simulink model "benign_PP"  (R2017a)
settings: Solver=FixedStepDiscrete  StartTime=0.0  StopTime=100  FixedStep=1  RelTol=1e-3
model workspace (MAT data in the model file):
  MCOS : class17 (value not decoded)
  compositionalMap : struct (value not decoded)
  isPreprocessedModel = 1
  MCOS : class17 (value not decoded)
  verificationResults : struct (value not decoded)
undefined symbols (not defined in the file or in its folder): contractAfterSimulation, contractBeforeSimulation, saveValidatorParameters
undefined symbols (not defined in the file): ContractBlock, ContractGuaranteeBlock, ContractValidatorBlock
libraries: simulink x436, CoCoSimSpecification x31
(part 3 of 3)

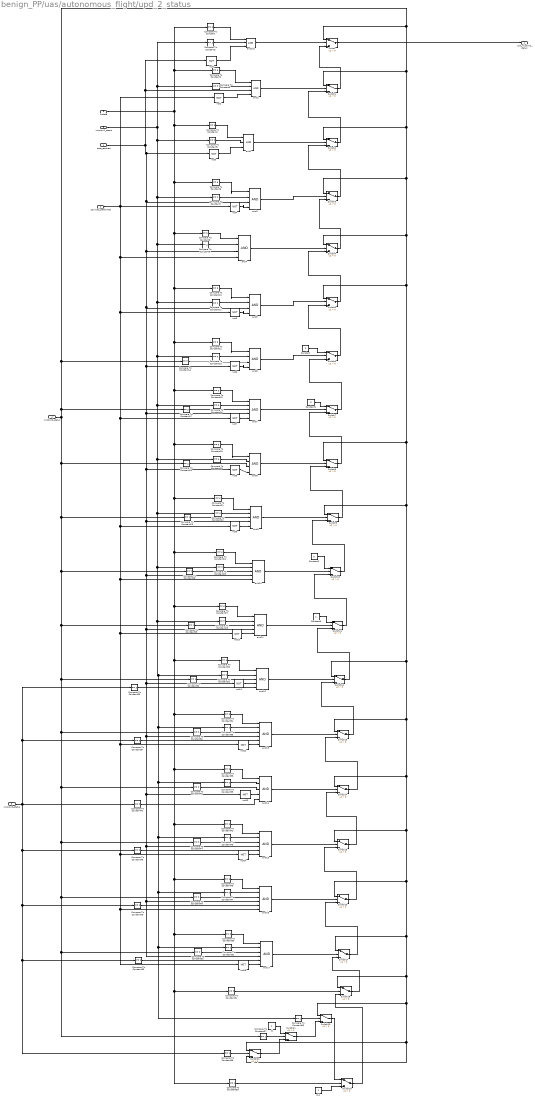
== system benign_PP/uas/autonomous_flight/upd_2_status ==
  dest_reached : Inport  OutDataTypeStr=boolean
  payload_performed : Inport  Port=2  OutDataTypeStr=boolean
  mission1_status : Inport  Port=3  OutDataTypeStr=int32
  mission2_status : Inport  Port=4  OutDataTypeStr=int32
  mission3_status : Inport  Port=5  OutDataTypeStr=int32
  mstate : Inport  Port=6  OutDataTypeStr=int32
  Compare To Constant{,2,4,6,8,10,12,15,18,21,24,27,30,34,38,42,46,50} (18 alike) : simulink/Logic and Bit Operations/Compare To Constant  relop===  const=6  OutDataTypeStr=boolean
  Compare To Constant{1,3,14,17,33,37,54} (7 alike) : simulink/Logic and Bit Operations/Compare To Constant  relop===  const=3  OutDataTypeStr=boolean
  Compare To Constant{5,7,9,11,20,23,26,29,41,45,49,53,56..58} (15 alike) : simulink/Logic and Bit Operations/Compare To Constant  relop===  const=2  OutDataTypeStr=boolean
  Compare To Constant{13,16,19,22,25,28,31..32,35..36,39..40,43..44,47..48,51..52} (18 alike) : simulink/Logic and Bit Operations/Compare To Constant  relop===  const=0  OutDataTypeStr=boolean
  Compare To Constant55 : simulink/Logic and Bit Operations/Compare To Constant  relop===  const=4  OutDataTypeStr=boolean
  Constant : Constant  Value=2  OutDataTypeStr=int32
  Constant1 : Constant  Value=2  OutDataTypeStr=int32
  Constant2 : Constant  Value=0  OutDataTypeStr=int32
  Constant3 : Constant  OutDataTypeStr=int32
  Switch{,2..22} (22 alike) : Switch  Criteria=u2 > Threshold
  Switch1 : Switch  Criteria=u2 > Threshold  OutDataTypeStr=int32
  and1 : Logic  Inputs=3  IconShape=distinctive  AllPortsSameDT=off  OutDataTypeStr=boolean
  and{7,9..12,14} (6 alike) : Logic  Inputs=5  IconShape=distinctive  AllPortsSameDT=off  OutDataTypeStr=boolean
  and101 : Logic  Inputs=3  IconShape=distinctive  AllPortsSameDT=off  OutDataTypeStr=boolean
  and{13,15..17} (4 alike) : Logic  Inputs=6  IconShape=distinctive  AllPortsSameDT=off  OutDataTypeStr=boolean
  and{2..6,8} (6 alike) : Logic  Inputs=4  IconShape=distinctive  AllPortsSameDT=off  OutDataTypeStr=boolean
  c1 : Constant  OutDataTypeStr=int32
  c11 : Constant  OutDataTypeStr=int32
  not{1..15} (15 alike) : Logic  Operator=NOT  Inputs=3  IconShape=distinctive  AllPortsSameDT=off  OutDataTypeStr=boolean
  upd_mission2_status : Outport  OutDataTypeStr=int32
  wires:
  c11/1 -> Switch19/3
  Switch/1 -> upd_mission2_status/1
  and101/1 -> Switch/2
  Compare To Constant/1 -> and101/1
  Compare To Constant1/1 -> and101/2
  not1/1 -> and101/3
  Compare To Constant3/1 -> and2/2
  Compare To Constant2/1 -> and2/1
  Switch1/1 -> Switch/3
  and2/1 -> Switch1/2
  not2/1 -> and2/4
  Switch2/1 -> Switch1/3
  Compare To Constant4/1 -> and1/1
  Compare To Constant5/1 -> and1/2
  and1/1 -> Switch2/2
  not3/1 -> and1/3
  and3/1 -> Switch3/2
  Compare To Constant7/1 -> and3/2
  Switch3/1 -> Switch2/3
  Compare To Constant6/1 -> and3/1
  not4/1 -> and3/4
  Compare To Constant8/1 -> and4/1
  and4/1 -> Switch4/2
  Compare To Constant9/1 -> and4/2
  Switch4/1 -> Switch3/3
  Compare To Constant10/1 -> and5/1
  Compare To Constant11/1 -> and5/2
  and5/1 -> Switch5/2
  not5/1 -> and5/4
  Switch5/1 -> Switch4/3
  Compare To Constant13/1 -> and6/2
  Compare To Constant12/1 -> and6/1
  not6/1 -> and6/4
  Switch6/1 -> Switch5/3
  and6/1 -> Switch6/2
  Compare To Constant14/1 -> and6/3
  Compare To Constant17/1 -> and7/3
  and7/1 -> Switch7/2
  Compare To Constant16/1 -> and7/2
  Compare To Constant15/1 -> and7/1
  Switch7/1 -> Switch6/3
  not7/1 -> and7/5
  Compare To Constant18/1 -> and8/1
  Compare To Constant20/1 -> and8/3
  and8/1 -> Switch8/2
  Switch8/1 -> Switch7/3
  Compare To Constant19/1 -> and8/2
  not8/1 -> and8/4
  Switch9/1 -> Switch8/3
  Compare To Constant21/1 -> and9/1
  Compare To Constant23/1 -> and9/3
  and9/1 -> Switch9/2
  Compare To Constant22/1 -> and9/2
  not9/1 -> and9/5
  Switch10/1 -> Switch9/3
  and10/1 -> Switch10/2
  Compare To Constant24/1 -> and10/1
  Compare To Constant26/1 -> and10/3
  Compare To Constant25/1 -> and10/2
  Switch11/1 -> Switch10/3
  Compare To Constant29/1 -> and11/3
  and11/1 -> Switch11/2
  Compare To Constant28/1 -> and11/2
  Compare To Constant27/1 -> and11/1
  not10/1 -> and11/5
  Compare To Constant30/1 -> and12/1
  Switch12/1 -> Switch11/3
  Compare To Constant31/1 -> and12/2
  and12/1 -> Switch12/2
  Compare To Constant32/1 -> and12/3
  not11/1 -> and12/4
  Compare To Constant33/1 -> and12/5
  Switch13/1 -> Switch12/3
  Compare To Constant37/1 -> and13/5
  and13/1 -> Switch13/2
  Compare To Constant34/1 -> and13/1
  Compare To Constant35/1 -> and13/2
  Compare To Constant36/1 -> and13/3
  not12/1 -> and13/6
  Compare To Constant40/1 -> and14/3
  Compare To Constant39/1 -> and14/2
  Compare To Constant38/1 -> and14/1
  Compare To Constant41/1 -> and14/5
  Switch14/1 -> Switch13/3
  and14/1 -> Switch14/2
  not13/1 -> and14/4
  and15/1 -> Switch15/2
  Compare To Constant45/1 -> and15/5
  Compare To Constant44/1 -> and15/3
  Switch15/1 -> Switch14/3
  not14/1 -> and15/6
  Compare To Constant42/1 -> and15/1
  Compare To Constant43/1 -> and15/2
  Switch16/1 -> Switch15/3
  Compare To Constant46/1 -> and16/1
  and16/1 -> Switch16/2
  Compare To Constant48/1 -> and16/3
  Compare To Constant47/1 -> and16/2
  Compare To Constant49/1 -> and16/5
  and17/1 -> Switch17/2
  Compare To Constant51/1 -> and17/2
  dest_reached/1 -> and2/3, not1/1, and9/4, and16/4, and17/4, and15/4, not13/1, and13/4, not11/1, and11/4, and10/4, not8/1, and7/4, not6/1, and5/3, and4/3, and3/3, not3/1
  Compare To Constant53/1 -> and17/5
  Compare To Constant50/1 -> and17/1
  mission1_status/1 -> Compare To Constant7/1, Compare To Constant56/1, Compare To Constant51/1, Compare To Constant47/1, Compare To Constant43/1, Compare To Constant39/1, Compare To Constant35/1, Compare To Constant31/1, Compare To Constant28/1, Compare To Constant25/1, Compare To Constant22/1, Compare To Constant19/1, Compare To Constant16/1, Compare To Constant13/1, Compare To Constant11/1, Compare To Constant9/1, Compare To Constant5/1, Compare To Constant3/1, Compare To Constant1/1
  Compare To Constant52/1 -> and17/3
  Switch17/1 -> Switch16/3
  not15/1 -> and17/6
  Switch18/1 -> Switch17/3
  Compare To Constant54/1 -> Switch18/2
  Switch19/1 -> Switch18/3
  mstate/1 -> Compare To Constant6/1, Compare To Constant12/1, Compare To Constant27/1, Compare To Constant55/1, Compare To Constant54/1, Compare To Constant50/1, Compare To Constant46/1, Compare To Constant42/1, Compare To Constant38/1, Compare To Constant34/1, Compare To Constant30/1, Compare To Constant24/1, Compare To Constant21/1, Compare To Constant18/1, Compare To Constant15/1, Compare To Constant10/1, Compare To Constant8/1, Compare To Constant4/1, Compare To Constant2/1, Compare To Constant/1
  Compare To Constant55/1 -> Switch19/2
  Compare To Constant56/1 -> Switch20/2
  mission2_status/1 -> Switch/1, Switch1/1, Switch2/1, Switch3/1, Switch4/1, Switch5/1, Switch8/1, Switch9/1, Switch12/1, Switch13/1, Switch14/1, Switch15/1, Switch16/1, Switch17/1, Switch18/1, Switch22/1, Switch22/3, Switch20/1, Compare To Constant14/1, Compare To Constant17/1, Compare To Constant57/1, Compare To Constant52/1, Compare To Constant48/1, Compare To Constant44/1, Compare To Constant40/1, Compare To Constant36/1, Compare To Constant32/1, Compare To Constant29/1, Compare To Constant26/1, Compare To Constant23/1, Compare To Constant20/1
  Switch20/1 -> Switch19/1
  Compare To Constant57/1 -> Switch21/2
  Switch21/1 -> Switch20/3
  Compare To Constant58/1 -> Switch22/2
  Switch22/1 -> Switch21/3
  mission3_status/1 -> Compare To Constant33/1, Compare To Constant37/1, Compare To Constant49/1, Compare To Constant58/1, Compare To Constant53/1, Compare To Constant45/1, Compare To Constant41/1
  payload_performed/1 -> not2/1, not15/1, and16/6, not14/1, not12/1, not10/1, and10/5, not9/1, not7/1, not5/1, and4/4, not4/1
  Constant1/1 -> Switch7/1
  Constant/1 -> Switch6/1
  Constant2/1 -> Switch10/1
  Constant3/1 -> Switch11/1
  c1/1 -> Switch21/1

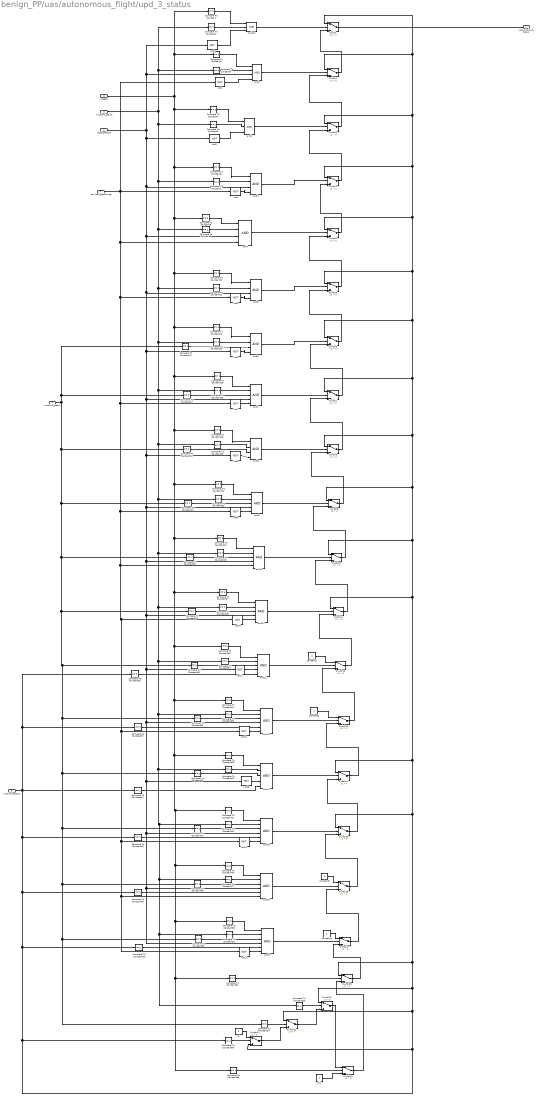
== system benign_PP/uas/autonomous_flight/upd_3_status ==
  dest_reached : Inport  OutDataTypeStr=boolean
  payload_performed : Inport  Port=2  OutDataTypeStr=boolean
  mission1_status : Inport  Port=3  OutDataTypeStr=int32
  mission2_status : Inport  Port=4  OutDataTypeStr=int32
  mission3_status : Inport  Port=5  OutDataTypeStr=int32
  mstate : Inport  Port=6  OutDataTypeStr=int32
  Compare To Constant{,2,4,6,8,10,12,15,18,21,24,27,30,34,38,42,46,50} (18 alike) : simulink/Logic and Bit Operations/Compare To Constant  relop===  const=6  OutDataTypeStr=boolean
  Compare To Constant{1,3,14,17,33,37,54} (7 alike) : simulink/Logic and Bit Operations/Compare To Constant  relop===  const=3  OutDataTypeStr=boolean
  Compare To Constant{5,7,9,11,20,23,26,29,41,45,49,53,56..58} (15 alike) : simulink/Logic and Bit Operations/Compare To Constant  relop===  const=2  OutDataTypeStr=boolean
  Compare To Constant{13,16,19,22,25,28,31..32,35..36,39..40,43..44,47..48,51..52} (18 alike) : simulink/Logic and Bit Operations/Compare To Constant  relop===  const=0  OutDataTypeStr=boolean
  Compare To Constant55 : simulink/Logic and Bit Operations/Compare To Constant  relop===  const=4  OutDataTypeStr=boolean
  Constant1 : Constant  Value=2  OutDataTypeStr=int32
  Constant2 : Constant  Value=2  OutDataTypeStr=int32
  Constant3 : Constant  Value=0  OutDataTypeStr=int32
  Constant4 : Constant  OutDataTypeStr=int32
  Switch : Switch  Criteria=u2 > Threshold  OutDataTypeStr=int32
  Switch{1..22} (22 alike) : Switch  Criteria=u2 > Threshold
  and1 : Logic  Inputs=3  IconShape=distinctive  AllPortsSameDT=off  OutDataTypeStr=boolean
  and{7,9..12,14} (6 alike) : Logic  Inputs=5  IconShape=distinctive  AllPortsSameDT=off  OutDataTypeStr=boolean
  and101 : Logic  Inputs=3  IconShape=distinctive  AllPortsSameDT=off  OutDataTypeStr=boolean
  and{13,15..17} (4 alike) : Logic  Inputs=6  IconShape=distinctive  AllPortsSameDT=off  OutDataTypeStr=boolean
  and{2..6,8} (6 alike) : Logic  Inputs=4  IconShape=distinctive  AllPortsSameDT=off  OutDataTypeStr=boolean
  c1 : Constant  OutDataTypeStr=int32
  c11 : Constant  OutDataTypeStr=int32
  not{1..15} (15 alike) : Logic  Operator=NOT  Inputs=3  IconShape=distinctive  AllPortsSameDT=off  OutDataTypeStr=boolean
  upd_mission3_status : Outport  OutDataTypeStr=int32
  wires:
  mission3_status/1 -> Compare To Constant41/1, Compare To Constant45/1, Compare To Constant53/1, Switch22/3, Switch21/1, Switch20/1, Switch18/1, Switch15/1, Switch14/1, Switch11/1, Switch10/1, Switch9/1, Switch8/1, Switch7/1, Switch6/1, Switch5/1, Switch4/1, Switch3/1, Switch2/1, Switch1/1, Switch/1, Compare To Constant58/1, Compare To Constant49/1, Compare To Constant37/1, Compare To Constant33/1
  payload_performed/1 -> not4/1, and4/4, not5/1, not7/1, not9/1, and10/5, not10/1, not12/1, not14/1, and16/6, not15/1, not2/1
  Switch22/1 -> Switch21/3
  Compare To Constant58/1 -> Switch22/2
  Switch21/1 -> Switch20/3
  Compare To Constant57/1 -> Switch21/2
  Switch20/1 -> Switch19/1
  mission2_status/1 -> Compare To Constant20/1, Compare To Constant23/1, Compare To Constant26/1, Compare To Constant29/1, Compare To Constant32/1, Compare To Constant36/1, Compare To Constant40/1, Compare To Constant44/1, Compare To Constant48/1, Compare To Constant52/1, Compare To Constant57/1, Compare To Constant17/1, Compare To Constant14/1
  Compare To Constant56/1 -> Switch20/2
  Compare To Constant55/1 -> Switch19/2
  mstate/1 -> Compare To Constant/1, Compare To Constant2/1, Compare To Constant4/1, Compare To Constant8/1, Compare To Constant10/1, Compare To Constant15/1, Compare To Constant18/1, Compare To Constant21/1, Compare To Constant24/1, Compare To Constant30/1, Compare To Constant34/1, Compare To Constant38/1, Compare To Constant42/1, Compare To Constant46/1, Compare To Constant50/1, Compare To Constant54/1, Compare To Constant55/1, Compare To Constant27/1, Compare To Constant12/1, Compare To Constant6/1
  Switch19/1 -> Switch18/3
  Compare To Constant54/1 -> Switch18/2
  Switch18/1 -> Switch17/3
  not15/1 -> and17/6
  Switch17/1 -> Switch16/3
  Compare To Constant52/1 -> and17/3
  mission1_status/1 -> Compare To Constant1/1, Compare To Constant3/1, Compare To Constant5/1, Compare To Constant9/1, Compare To Constant11/1, Compare To Constant13/1, Compare To Constant16/1, Compare To Constant19/1, Compare To Constant22/1, Compare To Constant25/1, Compare To Constant28/1, Compare To Constant31/1, Compare To Constant35/1, Compare To Constant39/1, Compare To Constant43/1, Compare To Constant47/1, Compare To Constant51/1, Compare To Constant56/1, Compare To Constant7/1
  Compare To Constant50/1 -> and17/1
  Compare To Constant53/1 -> and17/5
  dest_reached/1 -> not3/1, and3/3, and4/3, and5/3, not6/1, and7/4, not8/1, and10/4, and11/4, not11/1, and13/4, not13/1, and15/4, and17/4, and16/4, and9/4, not1/1, and2/3
  Compare To Constant51/1 -> and17/2
  and17/1 -> Switch17/2
  Compare To Constant49/1 -> and16/5
  Compare To Constant47/1 -> and16/2
  Compare To Constant48/1 -> and16/3
  and16/1 -> Switch16/2
  Compare To Constant46/1 -> and16/1
  Switch16/1 -> Switch15/3
  Compare To Constant43/1 -> and15/2
  Compare To Constant42/1 -> and15/1
  not14/1 -> and15/6
  Switch15/1 -> Switch14/3
  Compare To Constant44/1 -> and15/3
  Compare To Constant45/1 -> and15/5
  and15/1 -> Switch15/2
  not13/1 -> and14/4
  and14/1 -> Switch14/2
  Switch14/1 -> Switch13/3
  Compare To Constant41/1 -> and14/5
  Compare To Constant38/1 -> and14/1
  Compare To Constant39/1 -> and14/2
  Compare To Constant40/1 -> and14/3
  not12/1 -> and13/6
  Compare To Constant36/1 -> and13/3
  Compare To Constant35/1 -> and13/2
  Compare To Constant34/1 -> and13/1
  and13/1 -> Switch13/2
  Compare To Constant37/1 -> and13/5
  Switch13/1 -> Switch12/3
  Compare To Constant33/1 -> and12/5
  not11/1 -> and12/4
  Compare To Constant32/1 -> and12/3
  and12/1 -> Switch12/2
  Compare To Constant31/1 -> and12/2
  Switch12/1 -> Switch11/3
  Compare To Constant30/1 -> and12/1
  not10/1 -> and11/5
  Compare To Constant27/1 -> and11/1
  Compare To Constant28/1 -> and11/2
  and11/1 -> Switch11/2
  Compare To Constant29/1 -> and11/3
  Switch11/1 -> Switch10/3
  Compare To Constant25/1 -> and10/2
  Compare To Constant26/1 -> and10/3
  Compare To Constant24/1 -> and10/1
  and10/1 -> Switch10/2
  Switch10/1 -> Switch9/3
  not9/1 -> and9/5
  Compare To Constant22/1 -> and9/2
  and9/1 -> Switch9/2
  Compare To Constant23/1 -> and9/3
  Compare To Constant21/1 -> and9/1
  Switch9/1 -> Switch8/3
  not8/1 -> and8/4
  Compare To Constant19/1 -> and8/2
  Switch8/1 -> Switch7/3
  and8/1 -> Switch8/2
  Compare To Constant20/1 -> and8/3
  Compare To Constant18/1 -> and8/1
  not7/1 -> and7/5
  Switch7/1 -> Switch6/3
  Compare To Constant15/1 -> and7/1
  Compare To Constant16/1 -> and7/2
  and7/1 -> Switch7/2
  Compare To Constant17/1 -> and7/3
  Compare To Constant14/1 -> and6/3
  and6/1 -> Switch6/2
  Switch6/1 -> Switch5/3
  not6/1 -> and6/4
  Compare To Constant12/1 -> and6/1
  Compare To Constant13/1 -> and6/2
  Switch5/1 -> Switch4/3
  not5/1 -> and5/4
  and5/1 -> Switch5/2
  Compare To Constant11/1 -> and5/2
  Compare To Constant10/1 -> and5/1
  Switch4/1 -> Switch3/3
  Compare To Constant9/1 -> and4/2
  and4/1 -> Switch4/2
  Compare To Constant8/1 -> and4/1
  not4/1 -> and3/4
  Compare To Constant6/1 -> and3/1
  Switch3/1 -> Switch2/3
  Compare To Constant7/1 -> and3/2
  and3/1 -> Switch3/2
  not3/1 -> and1/3
  and1/1 -> Switch2/2
  Compare To Constant5/1 -> and1/2
  Compare To Constant4/1 -> and1/1
  Switch2/1 -> Switch1/3
  not2/1 -> and2/4
  and2/1 -> Switch1/2
  Switch1/1 -> Switch/3
  Compare To Constant2/1 -> and2/1
  Compare To Constant3/1 -> and2/2
  not1/1 -> and101/3
  Compare To Constant1/1 -> and101/2
  Compare To Constant/1 -> and101/1
  and101/1 -> Switch/2
  Switch/1 -> upd_mission3_status/1
  c11/1 -> Switch19/3
  Constant1/1 -> Switch12/1
  Constant2/1 -> Switch13/1
  Constant3/1 -> Switch16/1
  Constant4/1 -> Switch17/1
  c1/1 -> Switch22/1

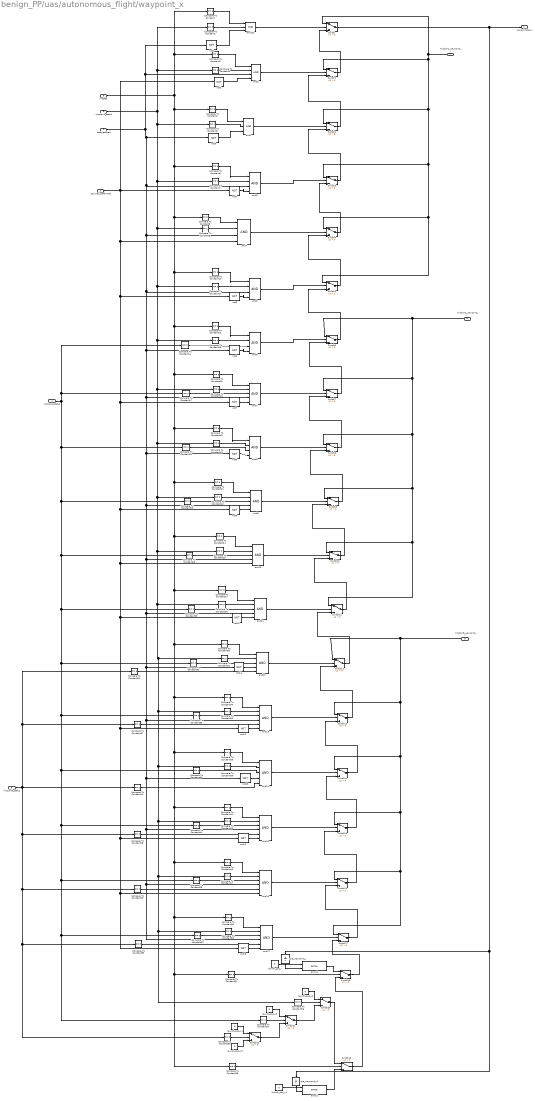
== system benign_PP/uas/autonomous_flight/waypoint_x ==
  dest_reached : Inport  OutDataTypeStr=boolean
  payload_performed : Inport  Port=2  OutDataTypeStr=boolean
  mission1_status : Inport  Port=3  OutDataTypeStr=int32
  mission2_status : Inport  Port=4  OutDataTypeStr=int32
  mission3_status : Inport  Port=5  OutDataTypeStr=int32
  mstate : Inport  Port=6  OutDataTypeStr=int32
  mission1_waypoint_x : Inport  Port=7  OutDataTypeStr=int32
  mission2_waypoint_x : Inport  Port=8  OutDataTypeStr=int32
  mission3_waypoint_x : Inport  Port=9  OutDataTypeStr=int32
  Compare To Constant{,2,4,6,8,10,12,15,18,21,24,27,30,34,38,42,46,50} (18 alike) : simulink/Logic and Bit Operations/Compare To Constant  relop===  const=6  OutDataTypeStr=boolean
  Compare To Constant{1,3,14,17,33,37,54} (7 alike) : simulink/Logic and Bit Operations/Compare To Constant  relop===  const=3  OutDataTypeStr=boolean
  Compare To Constant{5,7,9,11,20,23,26,29,41,45,49,53,56..58} (15 alike) : simulink/Logic and Bit Operations/Compare To Constant  relop===  const=2  OutDataTypeStr=boolean
  Compare To Constant{13,16,19,22,25,28,31..32,35..36,39..40,43..44,47..48,51..52} (18 alike) : simulink/Logic and Bit Operations/Compare To Constant  relop===  const=0  OutDataTypeStr=boolean
  Compare To Constant55 : simulink/Logic and Bit Operations/Compare To Constant  relop===  const=4  OutDataTypeStr=boolean
  Switch{,1..22} (23 alike) : Switch  Criteria=u2 > Threshold
  and1 : Logic  Inputs=3  IconShape=distinctive  AllPortsSameDT=off  OutDataTypeStr=boolean
  and{7,9..12,14} (6 alike) : Logic  Inputs=5  IconShape=distinctive  AllPortsSameDT=off  OutDataTypeStr=boolean
  and101 : Logic  Inputs=3  IconShape=distinctive  AllPortsSameDT=off  OutDataTypeStr=boolean
  and{13,15..17} (4 alike) : Logic  Inputs=6  IconShape=distinctive  AllPortsSameDT=off  OutDataTypeStr=boolean
  and{2..6,8} (6 alike) : Logic  Inputs=4  IconShape=distinctive  AllPortsSameDT=off  OutDataTypeStr=boolean
  arrow1 : CoCoSimSpecification/arrow  LustreOperatorBlock=ArrowOperator
      settings: SourceProductName=CoCoSim Specification
  arrow2 : CoCoSimSpecification/arrow  LustreOperatorBlock=ArrowOperator
      settings: SourceProductName=CoCoSim Specification
  launch_pos_x{,1..5} (6 alike) : Constant  Value=0  OutDataTypeStr=int32
  not{1..15} (15 alike) : Logic  Operator=NOT  Inputs=3  IconShape=distinctive  AllPortsSameDT=off  OutDataTypeStr=boolean
  pre_waypoint_x : UnitDelay  SampleTime=-1
  pre_waypoint_x1 : UnitDelay  SampleTime=-1
  waypointPos_x : Outport  OutDataTypeStr=int32
  wires:
  launch_pos_x5/1 -> Switch22/3
  mission3_status/1 -> Compare To Constant41/1, Compare To Constant45/1, Compare To Constant53/1, Compare To Constant58/1, Compare To Constant49/1, Compare To Constant37/1, Compare To Constant33/1
  launch_pos_x4/1 -> Switch22/1
  Switch22/1 -> Switch21/3
  Compare To Constant58/1 -> Switch22/2
  Switch21/1 -> Switch20/3
  Compare To Constant57/1 -> Switch21/2
  launch_pos_x3/1 -> Switch21/1
  Switch20/1 -> Switch19/1
  launch_pos_x2/1 -> Switch20/1
  Compare To Constant56/1 -> Switch20/2
  Compare To Constant55/1 -> Switch19/2
  mstate/1 -> Compare To Constant/1, Compare To Constant2/1, Compare To Constant4/1, Compare To Constant8/1, Compare To Constant10/1, Compare To Constant15/1, Compare To Constant18/1, Compare To Constant21/1, Compare To Constant24/1, Compare To Constant30/1, Compare To Constant34/1, Compare To Constant38/1, Compare To Constant42/1, Compare To Constant46/1, Compare To Constant50/1, Compare To Constant54/1, Compare To Constant55/1, Compare To Constant27/1, Compare To Constant12/1, Compare To Constant6/1
  Switch19/1 -> Switch18/3
  Compare To Constant54/1 -> Switch18/2
  Switch18/1 -> Switch17/3
  not15/1 -> and17/6
  Switch17/1 -> Switch16/3
  Compare To Constant52/1 -> and17/3
  mission1_status/1 -> Compare To Constant1/1, Compare To Constant3/1, Compare To Constant5/1, Compare To Constant9/1, Compare To Constant11/1, Compare To Constant13/1, Compare To Constant16/1, Compare To Constant19/1, Compare To Constant22/1, Compare To Constant25/1, Compare To Constant28/1, Compare To Constant31/1, Compare To Constant35/1, Compare To Constant39/1, Compare To Constant43/1, Compare To Constant47/1, Compare To Constant51/1, Compare To Constant56/1, Compare To Constant7/1
  Compare To Constant50/1 -> and17/1
  Compare To Constant53/1 -> and17/5
  dest_reached/1 -> not3/1, and3/3, and4/3, and5/3, not6/1, and7/4, not8/1, and10/4, and11/4, not11/1, and13/4, not13/1, and15/4, and17/4, and16/4, and9/4, not1/1, and2/3
  mission2_status/1 -> Compare To Constant20/1, Compare To Constant23/1, Compare To Constant26/1, Compare To Constant29/1, Compare To Constant32/1, Compare To Constant36/1, Compare To Constant40/1, Compare To Constant44/1, Compare To Constant48/1, Compare To Constant52/1, Compare To Constant57/1, Compare To Constant17/1, Compare To Constant14/1
  Compare To Constant51/1 -> and17/2
  payload_performed/1 -> not4/1, and4/4, not5/1, not7/1, not9/1, and10/5, not10/1, not12/1, not14/1, and16/6, not15/1, not2/1
  and17/1 -> Switch17/2
  Compare To Constant49/1 -> and16/5
  Compare To Constant47/1 -> and16/2
  Compare To Constant48/1 -> and16/3
  and16/1 -> Switch16/2
  Compare To Constant46/1 -> and16/1
  Switch16/1 -> Switch15/3
  Compare To Constant43/1 -> and15/2
  Compare To Constant42/1 -> and15/1
  not14/1 -> and15/6
  Switch15/1 -> Switch14/3
  Compare To Constant44/1 -> and15/3
  Compare To Constant45/1 -> and15/5
  and15/1 -> Switch15/2
  not13/1 -> and14/4
  and14/1 -> Switch14/2
  Switch14/1 -> Switch13/3
  Compare To Constant41/1 -> and14/5
  Compare To Constant38/1 -> and14/1
  Compare To Constant39/1 -> and14/2
  Compare To Constant40/1 -> and14/3
  not12/1 -> and13/6
  Compare To Constant36/1 -> and13/3
  Compare To Constant35/1 -> and13/2
  Compare To Constant34/1 -> and13/1
  and13/1 -> Switch13/2
  Compare To Constant37/1 -> and13/5
  Switch13/1 -> Switch12/3
  Compare To Constant33/1 -> and12/5
  not11/1 -> and12/4
  Compare To Constant32/1 -> and12/3
  and12/1 -> Switch12/2
  Compare To Constant31/1 -> and12/2
  Switch12/1 -> Switch11/3
  Compare To Constant30/1 -> and12/1
  not10/1 -> and11/5
  Compare To Constant27/1 -> and11/1
  Compare To Constant28/1 -> and11/2
  and11/1 -> Switch11/2
  Compare To Constant29/1 -> and11/3
  Switch11/1 -> Switch10/3
  Compare To Constant25/1 -> and10/2
  Compare To Constant26/1 -> and10/3
  Compare To Constant24/1 -> and10/1
  and10/1 -> Switch10/2
  Switch10/1 -> Switch9/3
  not9/1 -> and9/5
  Compare To Constant22/1 -> and9/2
  and9/1 -> Switch9/2
  Compare To Constant23/1 -> and9/3
  Compare To Constant21/1 -> and9/1
  Switch9/1 -> Switch8/3
  not8/1 -> and8/4
  Compare To Constant19/1 -> and8/2
  Switch8/1 -> Switch7/3
  and8/1 -> Switch8/2
  Compare To Constant20/1 -> and8/3
  Compare To Constant18/1 -> and8/1
  not7/1 -> and7/5
  Switch7/1 -> Switch6/3
  Compare To Constant15/1 -> and7/1
  Compare To Constant16/1 -> and7/2
  and7/1 -> Switch7/2
  Compare To Constant17/1 -> and7/3
  Compare To Constant14/1 -> and6/3
  and6/1 -> Switch6/2
  Switch6/1 -> Switch5/3
  not6/1 -> and6/4
  Compare To Constant12/1 -> and6/1
  Compare To Constant13/1 -> and6/2
  Switch5/1 -> Switch4/3
  not5/1 -> and5/4
  and5/1 -> Switch5/2
  Compare To Constant11/1 -> and5/2
  Compare To Constant10/1 -> and5/1
  Switch4/1 -> Switch3/3
  Compare To Constant9/1 -> and4/2
  and4/1 -> Switch4/2
  Compare To Constant8/1 -> and4/1
  not4/1 -> and3/4
  Compare To Constant6/1 -> and3/1
  Switch3/1 -> Switch2/3
  Compare To Constant7/1 -> and3/2
  and3/1 -> Switch3/2
  not3/1 -> and1/3
  and1/1 -> Switch2/2
  Compare To Constant5/1 -> and1/2
  Compare To Constant4/1 -> and1/1
  Switch2/1 -> Switch1/3
  not2/1 -> and2/4
  and2/1 -> Switch1/2
  Switch1/1 -> Switch/3
  Compare To Constant2/1 -> and2/1
  Compare To Constant3/1 -> and2/2
  not1/1 -> and101/3
  Compare To Constant1/1 -> and101/2
  Compare To Constant/1 -> and101/1
  and101/1 -> Switch/2
  mission1_waypoint_x/1 -> Switch1/1, Switch2/1, Switch3/1, Switch4/1, Switch5/1, Switch/1
  mission2_waypoint_x/1 -> Switch7/1, Switch8/1, Switch9/1, Switch10/1, Switch11/1, Switch6/1
  mission3_waypoint_x/1 -> Switch12/1, Switch13/1, Switch14/1, Switch15/1, Switch16/1, Switch17/1
  arrow1/1 -> Switch18/1
  launch_pos_x/1 -> arrow1/1
  launch_pos_x1/1 -> arrow2/1
  arrow2/1 -> Switch19/3
  Switch/1 -> pre_waypoint_x/1, pre_waypoint_x1/1, waypointPos_x/1
  pre_waypoint_x/1 -> arrow1/2
  pre_waypoint_x1/1 -> arrow2/2

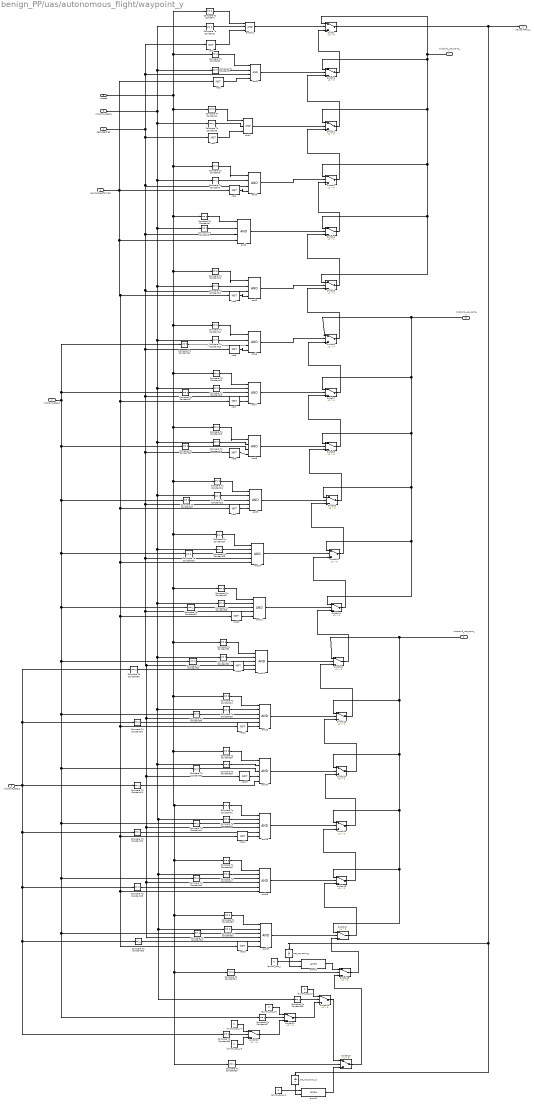
== system benign_PP/uas/autonomous_flight/waypoint_y ==
  dest_reached : Inport  OutDataTypeStr=boolean
  payload_performed : Inport  Port=2  OutDataTypeStr=boolean
  mission1_status : Inport  Port=3  OutDataTypeStr=int32
  mission2_status : Inport  Port=4  OutDataTypeStr=int32
  mission3_status : Inport  Port=5  OutDataTypeStr=int32
  mstate : Inport  Port=6  OutDataTypeStr=int32
  mission1_waypoint_y : Inport  Port=7  OutDataTypeStr=int32
  mission2_waypoint_y : Inport  Port=8  OutDataTypeStr=int32
  mission3_waypoint_y : Inport  Port=9  OutDataTypeStr=int32
  Compare To Constant{,2,4,6,8,10,12,15,18,21,24,27,30,34,38,42,46,50} (18 alike) : simulink/Logic and Bit Operations/Compare To Constant  relop===  const=6  OutDataTypeStr=boolean
  Compare To Constant{1,3,14,17,33,37,54} (7 alike) : simulink/Logic and Bit Operations/Compare To Constant  relop===  const=3  OutDataTypeStr=boolean
  Compare To Constant{5,7,9,11,20,23,26,29,41,45,49,53,56..58} (15 alike) : simulink/Logic and Bit Operations/Compare To Constant  relop===  const=2  OutDataTypeStr=boolean
  Compare To Constant{13,16,19,22,25,28,31..32,35..36,39..40,43..44,47..48,51..52} (18 alike) : simulink/Logic and Bit Operations/Compare To Constant  relop===  const=0  OutDataTypeStr=boolean
  Compare To Constant55 : simulink/Logic and Bit Operations/Compare To Constant  relop===  const=4  OutDataTypeStr=boolean
  Switch{,1..22} (23 alike) : Switch  Criteria=u2 > Threshold
  and1 : Logic  Inputs=3  IconShape=distinctive  AllPortsSameDT=off  OutDataTypeStr=boolean
  and{7,9..12,14} (6 alike) : Logic  Inputs=5  IconShape=distinctive  AllPortsSameDT=off  OutDataTypeStr=boolean
  "and101 " : Logic  Inputs=3  IconShape=distinctive  AllPortsSameDT=off  OutDataTypeStr=boolean
  and{13,15..17} (4 alike) : Logic  Inputs=6  IconShape=distinctive  AllPortsSameDT=off  OutDataTypeStr=boolean
  and{2..6,8} (6 alike) : Logic  Inputs=4  IconShape=distinctive  AllPortsSameDT=off  OutDataTypeStr=boolean
  arrow1 : CoCoSimSpecification/arrow  LustreOperatorBlock=ArrowOperator
      settings: SourceProductName=CoCoSim Specification
  arrow2 : CoCoSimSpecification/arrow  LustreOperatorBlock=ArrowOperator
      settings: SourceProductName=CoCoSim Specification
  launch_pos_y{,1..5} (6 alike) : Constant  Value=0  OutDataTypeStr=int32
  not{1..15} (15 alike) : Logic  Operator=NOT  Inputs=3  IconShape=distinctive  AllPortsSameDT=off  OutDataTypeStr=boolean
  pre_waypoint_y : UnitDelay  SampleTime=-1
  pre_waypoint_y1 : UnitDelay  SampleTime=-1
  waypointPos_y : Outport  OutDataTypeStr=int32
  wires:
  Switch/1 -> waypointPos_y/1, pre_waypoint_y1/1, pre_waypoint_y/1
  arrow2/1 -> Switch19/3
  launch_pos_y1/1 -> arrow2/1
  launch_pos_y/1 -> arrow1/1
  arrow1/1 -> Switch18/1
  mission3_waypoint_y/1 -> Switch17/1, Switch16/1, Switch15/1, Switch14/1, Switch13/1, Switch12/1
  mission2_waypoint_y/1 -> Switch6/1, Switch11/1, Switch10/1, Switch9/1, Switch8/1, Switch7/1
  mission1_waypoint_y/1 -> Switch/1, Switch5/1, Switch4/1, Switch3/1, Switch2/1, Switch1/1
  "and101 "/1 -> Switch/2
  Compare To Constant/1 -> "and101 "/1
  Compare To Constant1/1 -> "and101 "/2
  not1/1 -> "and101 "/3
  Compare To Constant3/1 -> and2/2
  Compare To Constant2/1 -> and2/1
  Switch1/1 -> Switch/3
  and2/1 -> Switch1/2
  not2/1 -> and2/4
  Switch2/1 -> Switch1/3
  Compare To Constant4/1 -> and1/1
  Compare To Constant5/1 -> and1/2
  and1/1 -> Switch2/2
  not3/1 -> and1/3
  and3/1 -> Switch3/2
  Compare To Constant7/1 -> and3/2
  Switch3/1 -> Switch2/3
  Compare To Constant6/1 -> and3/1
  not4/1 -> and3/4
  Compare To Constant8/1 -> and4/1
  and4/1 -> Switch4/2
  Compare To Constant9/1 -> and4/2
  Switch4/1 -> Switch3/3
  Compare To Constant10/1 -> and5/1
  Compare To Constant11/1 -> and5/2
  and5/1 -> Switch5/2
  not5/1 -> and5/4
  Switch5/1 -> Switch4/3
  Compare To Constant13/1 -> and6/2
  Compare To Constant12/1 -> and6/1
  not6/1 -> and6/4
  Switch6/1 -> Switch5/3
  and6/1 -> Switch6/2
  Compare To Constant14/1 -> and6/3
  Compare To Constant17/1 -> and7/3
  and7/1 -> Switch7/2
  Compare To Constant16/1 -> and7/2
  Compare To Constant15/1 -> and7/1
  Switch7/1 -> Switch6/3
  not7/1 -> and7/5
  Compare To Constant18/1 -> and8/1
  Compare To Constant20/1 -> and8/3
  and8/1 -> Switch8/2
  Switch8/1 -> Switch7/3
  Compare To Constant19/1 -> and8/2
  not8/1 -> and8/4
  Switch9/1 -> Switch8/3
  Compare To Constant21/1 -> and9/1
  Compare To Constant23/1 -> and9/3
  and9/1 -> Switch9/2
  Compare To Constant22/1 -> and9/2
  not9/1 -> and9/5
  Switch10/1 -> Switch9/3
  and10/1 -> Switch10/2
  Compare To Constant24/1 -> and10/1
  Compare To Constant26/1 -> and10/3
  Compare To Constant25/1 -> and10/2
  Switch11/1 -> Switch10/3
  Compare To Constant29/1 -> and11/3
  and11/1 -> Switch11/2
  Compare To Constant28/1 -> and11/2
  Compare To Constant27/1 -> and11/1
  not10/1 -> and11/5
  Compare To Constant30/1 -> and12/1
  Switch12/1 -> Switch11/3
  Compare To Constant31/1 -> and12/2
  and12/1 -> Switch12/2
  Compare To Constant32/1 -> and12/3
  not11/1 -> and12/4
  Compare To Constant33/1 -> and12/5
  Switch13/1 -> Switch12/3
  Compare To Constant37/1 -> and13/5
  and13/1 -> Switch13/2
  Compare To Constant34/1 -> and13/1
  Compare To Constant35/1 -> and13/2
  Compare To Constant36/1 -> and13/3
  not12/1 -> and13/6
  Compare To Constant40/1 -> and14/3
  Compare To Constant39/1 -> and14/2
  Compare To Constant38/1 -> and14/1
  Compare To Constant41/1 -> and14/5
  Switch14/1 -> Switch13/3
  and14/1 -> Switch14/2
  not13/1 -> and14/4
  and15/1 -> Switch15/2
  Compare To Constant45/1 -> and15/5
  Compare To Constant44/1 -> and15/3
  Switch15/1 -> Switch14/3
  not14/1 -> and15/6
  Compare To Constant42/1 -> and15/1
  Compare To Constant43/1 -> and15/2
  Switch16/1 -> Switch15/3
  Compare To Constant46/1 -> and16/1
  and16/1 -> Switch16/2
  Compare To Constant48/1 -> and16/3
  Compare To Constant47/1 -> and16/2
  Compare To Constant49/1 -> and16/5
  and17/1 -> Switch17/2
  payload_performed/1 -> not2/1, not15/1, and16/6, not14/1, not12/1, not10/1, and10/5, not9/1, not7/1, not5/1, and4/4, not4/1
  Compare To Constant51/1 -> and17/2
  mission2_status/1 -> Compare To Constant14/1, Compare To Constant17/1, Compare To Constant57/1, Compare To Constant52/1, Compare To Constant48/1, Compare To Constant44/1, Compare To Constant40/1, Compare To Constant36/1, Compare To Constant32/1, Compare To Constant29/1, Compare To Constant26/1, Compare To Constant23/1, Compare To Constant20/1
  dest_reached/1 -> and2/3, not1/1, and9/4, and16/4, and17/4, and15/4, not13/1, and13/4, not11/1, and11/4, and10/4, not8/1, and7/4, not6/1, and5/3, and4/3, and3/3, not3/1
  Compare To Constant53/1 -> and17/5
  Compare To Constant50/1 -> and17/1
  mission1_status/1 -> Compare To Constant7/1, Compare To Constant56/1, Compare To Constant51/1, Compare To Constant47/1, Compare To Constant43/1, Compare To Constant39/1, Compare To Constant35/1, Compare To Constant31/1, Compare To Constant28/1, Compare To Constant25/1, Compare To Constant22/1, Compare To Constant19/1, Compare To Constant16/1, Compare To Constant13/1, Compare To Constant11/1, Compare To Constant9/1, Compare To Constant5/1, Compare To Constant3/1, Compare To Constant1/1
  Compare To Constant52/1 -> and17/3
  Switch17/1 -> Switch16/3
  not15/1 -> and17/6
  Switch18/1 -> Switch17/3
  Compare To Constant54/1 -> Switch18/2
  Switch19/1 -> Switch18/3
  mstate/1 -> Compare To Constant6/1, Compare To Constant12/1, Compare To Constant27/1, Compare To Constant55/1, Compare To Constant54/1, Compare To Constant50/1, Compare To Constant46/1, Compare To Constant42/1, Compare To Constant38/1, Compare To Constant34/1, Compare To Constant30/1, Compare To Constant24/1, Compare To Constant21/1, Compare To Constant18/1, Compare To Constant15/1, Compare To Constant10/1, Compare To Constant8/1, Compare To Constant4/1, Compare To Constant2/1, Compare To Constant/1
  Compare To Constant55/1 -> Switch19/2
  Compare To Constant56/1 -> Switch20/2
  launch_pos_y2/1 -> Switch20/1
  Switch20/1 -> Switch19/1
  launch_pos_y3/1 -> Switch21/1
  Compare To Constant57/1 -> Switch21/2
  Switch21/1 -> Switch20/3
  Compare To Constant58/1 -> Switch22/2
  Switch22/1 -> Switch21/3
  launch_pos_y4/1 -> Switch22/1
  mission3_status/1 -> Compare To Constant33/1, Compare To Constant37/1, Compare To Constant49/1, Compare To Constant58/1, Compare To Constant53/1, Compare To Constant45/1, Compare To Constant41/1
  launch_pos_y5/1 -> Switch22/3
  pre_waypoint_y/1 -> arrow1/2
  pre_waypoint_y1/1 -> arrow2/2
